simulink model "Integrator"  (R2015b)
settings: Solver=VariableStepAuto  StartTime=0.0  StopTime=10.0  RelTol=1e-3
StartFcn:
  | open_scope
settings Model: Creator=LUBO  LastModifiedBy=LUBO

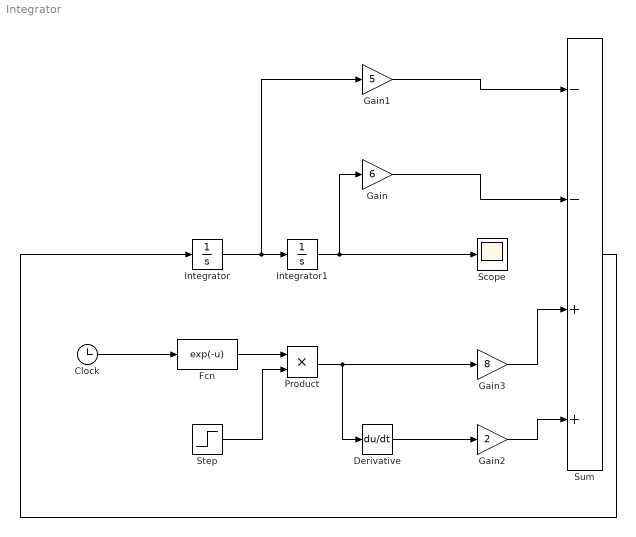
== system Integrator ==
  Clock : Clock
  Derivative : Derivative
  Fcn : Fcn  Expr=exp(-u)
  Gain : Gain  Gain=6
  Gain1 : Gain  Gain=5
  Gain2 : Gain  Gain=2
  Gain3 : Gain  Gain=8
  Integrator : Integrator  InitialCondition=-4
  Integrator1 : Integrator  InitialCondition=5
  Product : Product
  Scope : Scope
  Step : Step  SampleTime=0
  Sum : Sum  Inputs=--++
  wires:
  Clock/1 -> Fcn/1
  Fcn/1 -> Product/1
  Step/1 -> Product/2
  Product/1 -> Derivative/1, Gain3/1
  Derivative/1 -> Gain2/1
  Sum/1 -> Integrator/1
  Integrator/1 -> Gain1/1, Integrator1/1
  Integrator1/1 -> Gain/1, Scope/1
  Gain2/1 -> Sum/4
  Gain3/1 -> Sum/3
  Gain1/1 -> Sum/1
  Gain/1 -> Sum/2
